simulink model "zad61"  (R2023b)
settings: Solver=ode4  StartTime=0.0  StopTime=25  FixedStep=0.001  RelTol=1e-3
values from neighbouring files (symbols this model uses):
  Kp = Kp_set(i)    [zad61_Main.m]    (also in zad62_pendulum_Main.m = zeta(1))
settings Model: Creator=henry  LastModifiedBy=henry

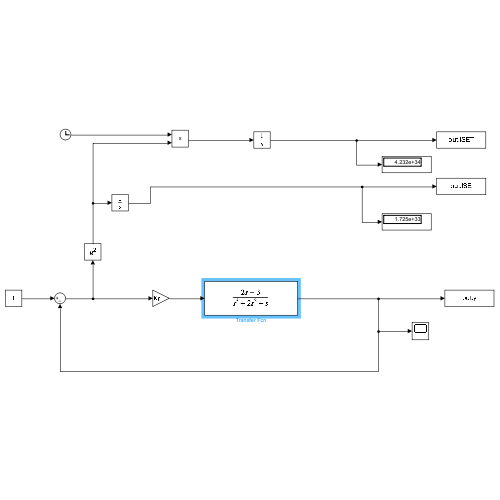
[thumbnail: Simulink's stored preview of the top-level diagram]
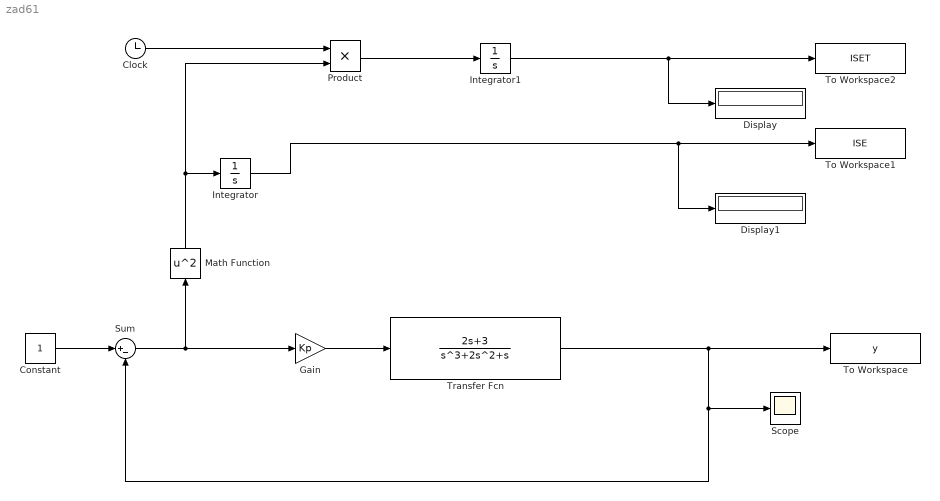
== system zad61 ==
  Clock : Clock
  Constant : Constant
  Display : Display
  Display1 : Display
  Gain : Gain  Gain=Kp
  Integrator : Integrator
  Integrator1 : Integrator
  Math Function : Math  Operator=square
  Product : Product
  Scope : Scope
  Sum : Sum  Inputs=|+-
  To Workspace : ToWorkspace  VariableName=y  SampleTime=-1
  To Workspace1 : ToWorkspace  VariableName=ISE  SampleTime=-1
  To Workspace2 : ToWorkspace  VariableName=ISET  SampleTime=-1
  Transfer Fcn : TransferFcn  Numerator=[0 0 2 3]  Denominator=[1 2 1 0]
  wires:
  Gain/1 -> Transfer Fcn/1
  Constant/1 -> Sum/1
  Sum/1 -> Gain/1, Math Function/1
  Transfer Fcn/1 -> Scope/1, Sum/2, To Workspace/1
  Integrator/1 -> Display1/1, To Workspace1/1
  Math Function/1 -> Product/2, Integrator/1
  Product/1 -> Integrator1/1
  Integrator1/1 -> Display/1, To Workspace2/1
  Clock/1 -> Product/1
